simulink model "PS_lab_Expt_5"  (R2015a)
settings: Solver=ode45  StartTime=0.0  StopTime=6  RelTol=1e-3
libraries: powerlib x9, dspstat3 x2, factslib x1
settings Model: Creator=student  LastModifiedBy=student

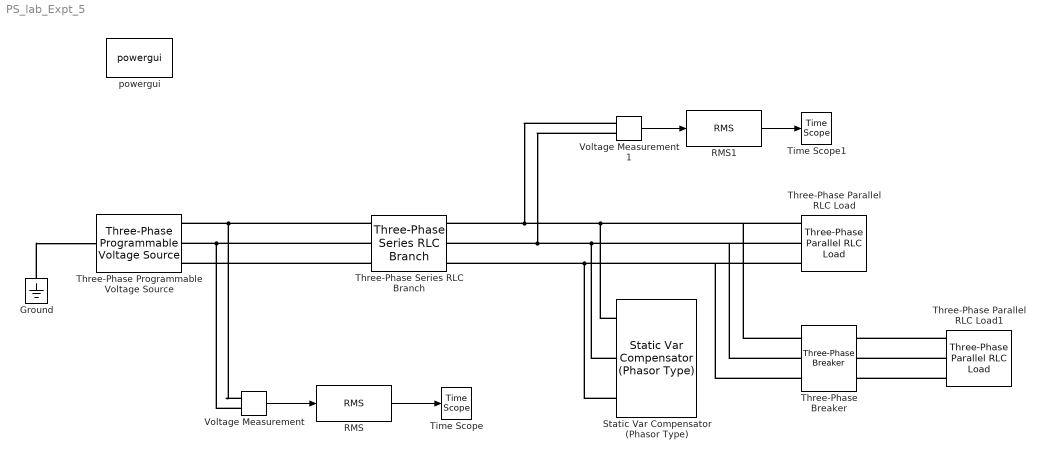
== system PS_lab_Expt_5 ==
  Ground : powerlib/Elements/Ground  LConnTagsString=a
  RMS : dspstat3/RMS  run=off  reset_popup=None  InputProcessing=Columns as channels (frame based)  directionMode=Each column  dimension=1  treatSBRowAsCol=off
  RMS1 : dspstat3/RMS  run=off  reset_popup=None  InputProcessing=Columns as channels (frame based)  directionMode=Each column  dimension=1  treatSBRowAsCol=off
  Static Var Compensator (Phasor Type) : factslib/Power-Electronics Based FACTS/Static Var Compensator (Phasor Type)  Seq1_Only=on  SystemNominal=[11e3, 50]  Pbase=10e6  Qnom="[200e4,  -200e4]"  Td=4e-3  mode=Voltage regulation  Vref=1.0  ExternalVref=off  Xs=0  Kp_Ki=[0 150]  Bref=0.0
  Three-Phase Parallel RLC Load : powerlib/Elements/Three-Phase Parallel RLC Load  LConnTagsString=A|B|C  Configuration=Y (grounded)  NominalVoltage=11e3  NominalFrequency=50  ActivePower=800e3  InductivePower=0  CapacitivePower=0  Measurements=None  LoadType=constant Z
  Three-Phase Parallel RLC Load1 : powerlib/Elements/Three-Phase Parallel RLC Load  LConnTagsString=A|B|C  Configuration=Y (grounded)  NominalVoltage=11e3  NominalFrequency=50  ActivePower=0  InductivePower=600e3  CapacitivePower=0  Measurements=None  LoadType=constant Z
  Three-Phase Programmable Voltage Source : powerlib/Electrical Sources/Three-Phase Programmable Voltage Source  PositiveSequence="[11e3  0 50]"  VariationEntity=Amplitude  VariationType=Table of time-amplitude pairs  VariationTypeAlt=Step  VariationStep=0.5  VariationRate=10  VariationMagnitude=0.3  VariationFrequency=2  VariationTiming=[1 2]  VariationPhaseA=off  Amplitudes=[1 0.95 1.05 1.0]  TimeValues=[0 1 2 3.5]  HarmonicGeneration=off  HarmonicA=[3 0.2 -25 0]  HarmonicB=[2 0.15 35 2]  Timing="[0.05  3]"  BusType=swing  Pref=0  Qref=0  Qmin=-inf  Qmax=inf
  Three-Phase Series RLC Branch : powerlib/Elements/Three-Phase Series RLC Branch  LConnTagsString=A|B|C  RConnTagsString=A|B|C  BranchType=RL  Resistance=.4  Inductance=4/314  Capacitance=1e-6  Measurements=None
  Three-Phase Breaker : powerlib/Elements/Three-Phase Breaker  InitialState=open  SwitchA=on  SwitchB=on  SwitchC=on  SwitchTimes=[3.5 5]  External=off  BreakerResistance=0.01  SnubberResistance=1e6  SnubberCapacitance=inf  Measurements=None
  Time Scope : TimeScope  DefaultConfigurationName=spbscopes.TimeScopeBlockCfg
  Time Scope1 : TimeScope  DefaultConfigurationName=spbscopes.TimeScopeBlockCfg
  Voltage Measurement : powerlib/Measurements/Voltage Measurement  PhasorSimulation=on  OutputType=Complex  PSBequivalent=0
  Voltage Measurement1 : powerlib/Measurements/Voltage Measurement  PhasorSimulation=on  OutputType=Complex  PSBequivalent=0
  powergui : powerlib/powergui  Priority=1  SimulationMode=Phasor  SolverType=Tustin/Backward Euler (TBE)  SampleTime=50e-6  frequency=50  SPID=off  DisableSnubberDevices=off  DisableRonSwitches=off  DisableVfSwitches=off  SwTol=0  DisplayEquations=off  Interpol=off  methode=off  Ts=100  FunctionMessages=off  echomessages=off  HookPort=off  EnableUseOfTLC=off  x0status=blocks  frequencyindice=50  Pbase=100e6  ErrMax=1e-4  Iterations=50  UnitsV=kV  UnitsW=MW  buscounter=0  RestoreLinks=warning  ResistiveCurrentMeasurement=off  Frange=[0:2:500]  Ylog=off  Xlog=on  ShowGrid=off  save=off  variable=ZData  structure=0  ZoomFFT=off  StartTime=0.0  cycles=1  DisplayStyle=1  fundamental=60  FreqAxis=off  MaxFrequency=1000  frequencyindicesteady=1  RmsSteady=1  display=off
  wires:
  Voltage Measurement/1 -> RMS/1
  RMS/1 -> Time Scope/1
  Voltage Measurement1/1 -> RMS1/1
  RMS1/1 -> Time Scope1/1
  connections:
  Three-Phase Series RLC Branch/LConn1 -- Voltage Measurement/LConn1 -- Three-Phase Programmable Voltage Source/RConn1
  Three-Phase Series RLC Branch/LConn2 -- Voltage Measurement/LConn2 -- Three-Phase Programmable Voltage Source/RConn2
  Three-Phase Series RLC Branch/LConn3 -- Three-Phase Programmable Voltage Source/RConn3
  Three-Phase Parallel RLC Load/LConn1 -- Three-Phase Breaker/LConn1 -- Voltage Measurement1/LConn1 -- Three-Phase Series RLC Branch/RConn1 -- Static Var Compensator (Phasor Type)/LConn1
  Three-Phase Parallel RLC Load/LConn2 -- Three-Phase Breaker/LConn2 -- Static Var Compensator (Phasor Type)/LConn2 -- Voltage Measurement1/LConn2 -- Three-Phase Series RLC Branch/RConn2
  Three-Phase Parallel RLC Load/LConn3 -- Three-Phase Breaker/LConn3 -- Static Var Compensator (Phasor Type)/LConn3 -- Three-Phase Series RLC Branch/RConn3
  Three-Phase Parallel RLC Load1/LConn1 -- Three-Phase Breaker/RConn1
  Three-Phase Parallel RLC Load1/LConn2 -- Three-Phase Breaker/RConn2
  Three-Phase Parallel RLC Load1/LConn3 -- Three-Phase Breaker/RConn3
  Ground/LConn1 -- Three-Phase Programmable Voltage Source/LConn1
